simulink model "blink_led_simu"  (R2023b)
settings: Solver=ode1  StartTime=0.0  StopTime=inf  FixedStep=1e-3  RelTol=1e-3  EnableMultiTasking=on
libraries: stm32f4xxblockslib x2, stm32blockslib x1, stm32f7xxblockslib x1
settings Model: STM32="{\"DigitalPortWrite\":{\"ID\":\"blink_led_simu:4\"},\"EncoderBlock\":[{\"ID\":\"blink_led_simu:7\"},{\"ID\":\"blink_led_simu:17\"}],\"AnalogInput\":{\"ID\":\"blink_led_simu:29\"},\"PWMOutput\":{\"ID\":\"blink_led_simu:31\"}}"  Creator=HP  LastModifiedBy=HP
settings SolverCC: AutoInsertRateTranBlk=on
settings OptimizationCC: EnhancedBackFolding=on  PassReuseOutputArgsAs=Individual arguments  ZeroExternalMemoryAtStartup=off  ZeroInternalMemoryAtStartup=off  MaxStackSize=64  OptimizeBlockOrder=speed  DifferentSizesBufferReuse=on  OptimizationCustomize=off  EfficientTunableParamExpr=on
settings DebuggingCC: ParameterTunabilityLossMsg=error
settings HardwareCC: ProdBitPerPointer=32  ProdBitPerSizeT=32  ProdBitPerPtrDiffT=32  ProdLargestAtomicInteger=Long  ProdLargestAtomicFloat=Double  ProdWordSize=32  ProdLongLongMode=on  ProdHWDeviceType=ARM Compatible->ARM Cortex
settings SFSimCC: MATLABDynamicMemAlloc=off
settings RTWCC: Description=Embedded Coder  SystemTargetFile=ert.tlc  HardwareBoard=STM32F7xx Based (Double precision FPU)  TemplateMakefile=ert_default_tmf  Toolchain=GNU Tools for ARM Embedded Processors
settings CodeAppCC: ForceParamTrailComments=on  IgnoreCustomStorageClasses=off  OperatorAnnotations=on  SimulinkDataObjDesc=on  SFDataObjDesc=on  InsertBlockDesc=on
settings ERTTargetCC: CodeReplacementLibrary=ARM Cortex-M  ExtModeTransport=3  ExtModeStaticAlloc=on  ExtModeStaticAllocSize=2048  ExtModeMexFile=ext_xcp  ExtModeIntrfLevel=Level2 - Open

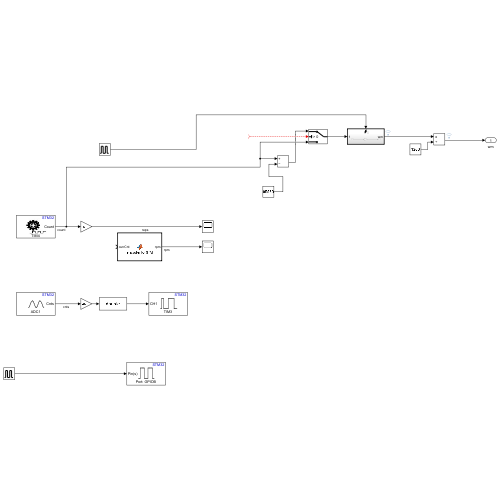
[thumbnail: Simulink's stored preview of the top-level diagram]
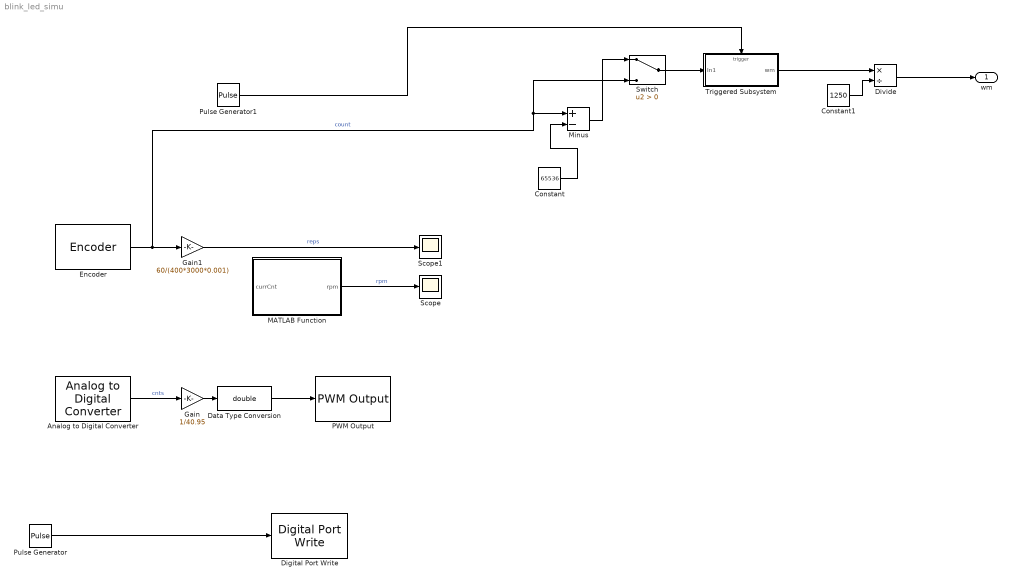
== system blink_led_simu ==
  Analog to Digital Converter : stm32f4xxblockslib/Analog to Digital Converter  ADCModule=ADC1  ConversionGroup=Regular  TriggerMode=Trigger and read  NumberOfConversions=1  EnableBufferConv=off  BufferLength=1  OutputStatus=off  SampleTime=-1  EnableSimPort=off  hoistedMaskSrc=ECSoC/ECSimCodegen/Analog to Digital Converter
      settings: LibrarySourceBlock=stm32f7xxblockslib/Analog to Digital Converter
  Constant : Constant  Value=65536
  Constant1 : Constant  Value=1250
  Data Type Conversion : DataTypeConversion  OutDataTypeStr=double  SaturateOnIntegerOverflow=off  RndMeth=Floor
  Digital Port Write : stm32f4xxblockslib/Digital Port Write  PortName=GPIOB  PinNumber=[0]  ReadOperation=off  IOAsArray=on  EnableSimPort=off  hoistedMaskSrc=ECSoC/ECSimCodegen/Digital Port Write
      settings: LibrarySourceBlock=stm32f7xxblockslib/Digital Port Write
  Divide : Product  Inputs=*/
  Encoder : stm32blockslib/Encoder  TimerModule=TIM4  EnableResetInput=off  OutputDirection=off  SampleTime=-1
      settings: LibrarySourceBlock=stm32f7xxblockslib/Encoder
  Gain : Gain  Gain=1/40.95
  Gain1 : Gain  Gain=60/(400*3000*0.001)
  MATLAB Function : MATLAB Function  TreatAsAtomicUnit=on
  Minus : Sum  Inputs=+-
  PWM Output : stm32f7xxblockslib/PWM Output  TimerModule=TIM3  DutycycleUnits=Percentage  EnableChannel1=on  EnableChannel2=off  EnableChannel3=off  EnableChannel4=off  EnableChannel5=off  EnableChannel6=off  EnableCounterInput=off  EnableMainOutputInput=off  EnableFrequencyInput=off  SetRCAfterCE=off  OutputDirection=off  OutputMainOutputEnableStatus=off  SampleTime=0.1  EnableSimPort=off  EnableUpdateEvent=off  EnableCaptureCompare1Event=off  EnableCaptureCompare2Event=off  EnableCaptureCompare3Event=off  EnableCaptureCompare4Event=off  EnableTriggerEvent=off  EnableBreakEvent=off  EnableBreakEvent2=off  ProcessorFamily=STM32F7  hoistedMaskSrc=ECSoC/ECSimCodegen/PWM Output
  Pulse Generator : DiscretePulseGenerator  PulseType=Time based  Period=10  PulseWidth=50
  Pulse Generator1 : DiscretePulseGenerator  PulseType=Time based  Period=0.01  PulseWidth=10
  Scope : Scope
  Scope1 : Scope
  Switch : Switch  Criteria=u2 > Threshold  SaturateOnIntegerOverflow=off  InputSameDT=off
  Triggered Subsystem : Subsystem  TreatAsAtomicUnit=on
  wm : Outport
  wires:
  Pulse Generator/1 -> Digital Port Write/1
  Analog to Digital Converter/1 -> Gain/1  "cnts"
  Gain/1 -> Data Type Conversion/1
  Data Type Conversion/1 -> PWM Output/1
  Encoder/1 -> Switch/3, Minus/1, Gain1/1  "count"
  MATLAB Function/1(rpm) -> Scope/1  "rpm"
  Gain1/1 -> Scope1/1  "reps"
  Constant/1 -> Minus/2
  Pulse Generator1/1 -> Triggered Subsystem/Trigger
  Switch/1 -> Triggered Subsystem/1(In1)
  Triggered Subsystem/1(wm) -> Divide/1
  Minus/1 -> Switch/1
  Constant1/1 -> Divide/2
  Divide/1 -> wm/1
  ? -> Switch/2

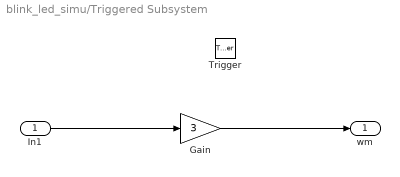
== system blink_led_simu/Triggered Subsystem ==
  In1 : Inport
  Trigger : TriggerPort  VariantControl=(inherit)
  Gain : Gain  Gain=3
  wm : Outport
  wires:
  In1/1 -> Gain/1
  Gain/1 -> wm/1

== matlab function blink_led_simu/MATLAB Function ==
  data: currCnt input; rpm output
function rpm = encoderToRPM(currCnt)
persistent prevCnt inited
if isempty(inited)
    prevCnt = int32(currCnt);
    inited = true;
    rpm = 0.0;
    return;
end

% 1) różnica z korekcją zawinięcia 16-bit
curr = int32(currCnt);
diff = curr - prevCnt;
if diff > 32767
    diff = diff - 65536;
elseif diff < -32768
    diff = diff + 65536;
end
prevCnt = curr;

% 2) parametry
dt = 0.001;         
PPR = 800;            
pulses_per_rev = PPR * 4;   % x4 w trybie TI1+TI2

% 3) RPM
revs_per_sec = double(diff) / double(pulses_per_rev) / dt;
rpm = revs_per_sec * 60.0;
end
